simulink library "vmc"  (R2021b)
settings: Solver=VariableStepAuto  StartTime=0.0  StopTime=10.0  RelTol=1e-3
undefined symbols (not defined in the file or in its folder): AVMC_ACCDeltaTqIGain4OVRD_X_kph, AVMC_ACCDeltaTqIGain4OVRD_Y_mps2, AVMC_ACCDeltaTqIGain_X_kph, AVMC_ACCDeltaTqIGain_Y_mps2, AVMC_ACCDeltaTqPGain_X_kph, AVMC_ACCDeltaTqPGain_Y_kph, AVMC_ACCLongSteadyCtrl_X_kph, AVMC_ADSPosGFBDeltaTq_X_kph, AVMC_ADSPosGFBDeltaTq_Y_mps2, AVMC_AggressJerkPCT4AT_X_kph, AVMC_AggressJerkPCT_X_kph, AVMC_AggressLimitPCT4AT_X_kph, AVMC_AggressLimitPCT_X_kph, AVMC_CCLongSteadyCtrl_X_kph, AVMC_DISCDeltaTqIGain_X_kph, AVMC_DISCDeltaTqIGain_Y_mps2, AVMC_DISCDeltaTqPGain_X_kph, AVMC_DISCDeltaTqPGain_Y_kph, AVMC_ESCRegenOut_X_kph, AVMC_ESCRegenOut_Y_Deg, AVMC_ESCRegenOutEnSpd_X_Deg, AVMC_ISOAccLimit_X_mps, AVMC_ISODecLimit_X_mps, AVMC_ISOJerk_X_mps, AVMC_LatESCRegenOut_X_kph, AVMC_LatESCRegenOut_Y_Deg, AVMC_LongAccDeadZone_X_kph, AVMC_LongAccFiltTsforP2_X_Gps, AVMC_MCPresBaseTq_X_bar, AVMC_MSALongSteadyCtrl_X_kph, AVMC_MSAPedalOvrd_X_kph, AVMC_MSASpdBand_X_kph, AVMC_MSATqDownEndTq_X_kph, AVMC_MSATqDownTime_X_kph, AVMC_OPDDisSlideRate_X_Deg, AVMC_OVRD2ActSR2FCMCMD_X_mps2, AVMC_PedalTqRWhlRatio_X_Nm, AVMC_PedalTqRWhlRatio_Y_gps, AVMC_PedalTqRWhlSlipGain_X_rat, AVMC_PedalTqRWhlSlipGain_Y_kph, AVMC_PedalTqRWhSTRGGain_X_deg, AVMC_PedalTqRWhSTRGGain_Y_kph, AVMC_RDCDetectTime_X_kph, AVMC_RDCDetectTime_Y_pct, AVMC_RDCEnSlideRate_X_Deg, AVMC_RearWhlTqRatio_X_Nm, AVMC_RearWhlTqRatio_Y_gps, AVMC_RearWhlTqSlipGain_X_rat, AVMC_RearWhlTqSlipGain_Y_kph, AVMC_RearWhlTqSTRGGain_X_deg, AVMC_RearWhlTqSTRGGain_Y_kph, AVMC_ReqBrkJoinDecSR_X_mps2, AVMC_SoftJerkPCT_X_kph, AVMC_SoftLimitPCT_X_kph, AVMC_StESCYaw_X_kph, AVMC_StESCYaw_Y_Deg, AVMC_StESCYawCom_X_kph, AVMC_StESCYawCom_Y_Gps, AVMC_TMSpdBaseTq_X_rpm, AVMC_VehHoldDecCtrlTime2_X_kph ... (+411)
libraries: hcu_lib x108, simulink x82, tqr x1, simulink_extras x1
(part 5 of 14)

== system vmc/VMC/VMC/Slide Rate  Calculation ==
  VINP_LFRawWhlSpeed_kph : Inport
  VINP_RFRawWhlSpeed_kph : Inport  Port=2
  VINP_LRRawWhlSpeed_kph : Inport  Port=3
  VINP_RRRawWhlSpeed_kph : Inport  Port=4
  VINP_VehSpeed_kph : Inport  Port=5
  VINP_BrkPedalPos_pct : Inport  Port=6
  VINP_BrkSwSta_flg : Inport  Port=7
  VINP_LongAccel_Gps : Inport  Port=8
  VVMC_LongAcc_Gps : Inport  Port=9
  task_time_s : Inport  Port=10
  VTQD_AfterAvailableTqDemFr_Nm : Inport  Port=11
  VTQD_AfterAvailableTqDemRr_Nm : Inport  Port=12
  VTQD_EquivAccPedalSWSta_flg : Inport  Port=13
  VTQD_GearActualPosn_enum : Inport  Port=14
  VTQD_RegenMode_enum : Inport  Port=15
  VTQD_VehActSpd_kph : Inport  Port=16
  VVMC_EstSlope_Deg : Inport  Port=17
  4Wheel Calculation : Subsystem
  Alternative Wheel Slide Calculation : Subsystem
  Coordination : Subsystem
  Partial Wheel Calculation : Subsystem
  VVMC_RawWhlSpdSlideRate_pct : Outport
  VVMC_LFWhlSpdSlideRate_pct : Outport  Port=2
  VVMC_RFWhlSpdSlideRate_pct : Outport  Port=3
  VVMC_LRWhlSpdSlideRate_pct : Outport  Port=4
  VVMC_RRWhlSpdSlideRate_pct : Outport  Port=5
  VVMC_LF4WhlSpdSlideRate_pct : Outport  Port=6
  VVMC_RF4WhlSpdSlideRate_pct : Outport  Port=7
  VVMC_LR4WhlSpdSlideRate_pct : Outport  Port=8
  VVMC_RR4WhlSpdSlideRate_pct : Outport  Port=9
  VVMC_PredictVehSpd_kph : Outport  Port=10
  VVMC_4WhlSpdSlideRate_pct : Outport  Port=11
  VVMC_ActMaxSlideRate_pct : Outport  Port=12
  VVMC_ActLFSlideRate_pct : Outport  Port=13
  VVMC_ActRFSlideRate_pct : Outport  Port=14
  VVMC_ActLRSlideRate_pct : Outport  Port=15
  VVMC_ActRRSlideRate_pct : Outport  Port=16
  VVMC_AltLWhlSlideRate_pct : Outport  Port=17
  VVMC_AltRWhlSlideRate_pct : Outport  Port=18
  VVMC_AltWhlSlideRate_pct : Outport  Port=19
  wires:
  VINP_BrkSwSta_flg/1 -> [VINP_BrkSwSta_flg]
  VTQD_AfterAvailableTqDemFr_Nm/1 -> [VTQD_AfterAvailableTqDemFr_Nm]
  [VVMC_RF4WhlSpdSlideRate_pct] -> VVMC_RF4WhlSpdSlideRate_pct/1
  [VVMC_ActRRSlideRate_pct] -> VVMC_ActRRSlideRate_pct/1
  VTQD_EquivAccPedalSWSta_flg/1 -> [VTQD_EquivAccPedalSWSta_flg]
  [VVMC_LFWhlSpdSlideRate_pct] -> VVMC_LFWhlSpdSlideRate_pct/1
  VINP_BrkPedalPos_pct/1 -> [VINP_BrkPedalPos_pct]
  [VVMC_RRWhlSpdSlideRate_pct] -> VVMC_RRWhlSpdSlideRate_pct/1
  task_time_s/1 -> [task_time_s]
  VINP_RRRawWhlSpeed_kph/1 -> [VINP_RRRawWhlSpeed_kph]
  [VVMC_ActMaxSlideRate_pct] -> VVMC_ActMaxSlideRate_pct/1
  [VVMC_RFWhlSpdSlideRate_pct] -> VVMC_RFWhlSpdSlideRate_pct/1
  [VVMC_LR4WhlSpdSlideRate_pct] -> VVMC_LR4WhlSpdSlideRate_pct/1
  [VVMC_ActRFSlideRate_pct] -> VVMC_ActRFSlideRate_pct/1
  [VVMC_RR4WhlSpdSlideRate_pct] -> VVMC_RR4WhlSpdSlideRate_pct/1
  VINP_RFRawWhlSpeed_kph/1 -> [VINP_RFRawWhlSpeed_kph]
  VINP_VehSpeed_kph/1 -> [VINP_VehSpeed_kph]
  [VVMC_ActLRSlideRate_pct] -> VVMC_ActLRSlideRate_pct/1
  [VVMC_PredictVehSpd_kph] -> VVMC_PredictVehSpd_kph/1
  VINP_LRRawWhlSpeed_kph/1 -> [VINP_LRRawWhlSpeed_kph]
  [VVMC_LF4WhlSpdSlideRate_pct] -> VVMC_LF4WhlSpdSlideRate_pct/1
  [VVMC_RawWhlSpdSlideRate_pct] -> VVMC_RawWhlSpdSlideRate_pct/1
  VINP_LFRawWhlSpeed_kph/1 -> [VINP_LFRawWhlSpeed_kph]
  [VVMC_LRWhlSpdSlideRate_pct] -> VVMC_LRWhlSpdSlideRate_pct/1
  [VVMC_ActLFSlideRate_pct] -> VVMC_ActLFSlideRate_pct/1
  [VVMC_4WhlSpdSlideRate_pct] -> VVMC_4WhlSpdSlideRate_pct/1
  VVMC_LongAcc_Gps/1 -> [VVMC_LongAcc_Gps]
  VTQD_AfterAvailableTqDemRr_Nm/1 -> [VTQD_AfterAvailableTqDemRr_Nm]
  [VINP_LFRawWhlSpeed_kph] -> Alternative Wheel Slide Calculation/1(VINP_LFRawWhlSpeed_kph)
  [VINP_RFRawWhlSpeed_kph] -> Alternative Wheel Slide Calculation/2(VINP_RFRawWhlSpeed_kph)
  [VINP_LRRawWhlSpeed_kph] -> Alternative Wheel Slide Calculation/3(VINP_LRRawWhlSpeed_kph)
  [VINP_RRRawWhlSpeed_kph] -> Alternative Wheel Slide Calculation/4(VINP_RRRawWhlSpeed_kph)
  Alternative Wheel Slide Calculation/1(VVMC_AltLWhlSlideRate_pct) -> [VVMC_AltLWhlSlideRate_pct]
  Alternative Wheel Slide Calculation/2(VVMC_AltRWhlSlideRate_pct) -> [VVMC_AltRWhlSlideRate_pct]
  Alternative Wheel Slide Calculation/3(VVMC_AltWhlSlideRate_pct) -> [VVMC_AltWhlSlideRate_pct]
  [VVMC_AltLWhlSlideRate_pct] -> VVMC_AltLWhlSlideRate_pct/1
  [VVMC_AltRWhlSlideRate_pct] -> VVMC_AltRWhlSlideRate_pct/1
  [VVMC_AltWhlSlideRate_pct] -> VVMC_AltWhlSlideRate_pct/1
  Partial Wheel Calculation/2(VVMC_LFWhlSpdSlideRate_pct) -> [VVMC_LFWhlSpdSlideRate_pct]
  Partial Wheel Calculation/5(VVMC_RRWhlSpdSlideRate_pct) -> [VVMC_RRWhlSpdSlideRate_pct]
  Partial Wheel Calculation/3(VVMC_RFWhlSpdSlideRate_pct) -> [VVMC_RFWhlSpdSlideRate_pct]
  Partial Wheel Calculation/1(VVMC_RawWhlSpdSlideRate_pct) -> [VVMC_RawWhlSpdSlideRate_pct]
  [VINP_RFRawWhlSpeed_kph] -> Partial Wheel Calculation/2(VINP_RFRawWhlSpeed_kph)
  [VINP_LRRawWhlSpeed_kph] -> Partial Wheel Calculation/3(VINP_LRRawWhlSpeed_kph)
  [VTQD_AfterAvailableTqDemFr_Nm] -> Partial Wheel Calculation/5(VTQD_AfterAvailableTqDemFr_Nm)
  [VINP_LFRawWhlSpeed_kph] -> Partial Wheel Calculation/1(VINP_LFRawWhlSpeed_kph)
  [VINP_RRRawWhlSpeed_kph] -> Partial Wheel Calculation/4(VINP_RRRawWhlSpeed_kph)
  [VTQD_AfterAvailableTqDemRr_Nm] -> Partial Wheel Calculation/6(VTQD_AfterAvailableTqDemRr_Nm)
  Partial Wheel Calculation/4(VVMC_LRWhlSpdSlideRate_pct) -> [VVMC_LRWhlSpdSlideRate_pct]
  4Wheel Calculation/3(VVMC_LR4WhlSpdSlideRate_pct) -> [VVMC_LR4WhlSpdSlideRate_pct]
  [task_time_s] -> 4Wheel Calculation/6(task_time_s)
  4Wheel Calculation/1(VVMC_LF4WhlSpdSlideRate_pct) -> [VVMC_LF4WhlSpdSlideRate_pct]
  4Wheel Calculation/7(VVMC_AllWhlSkid_flg) -> [VVMC_AllWhlSkid_flg]
  [VVMC_LongAcc_Gps] -> 4Wheel Calculation/5(VVMC_LongAcc_Gps)
  4Wheel Calculation/4(VVMC_RR4WhlSpdSlideRate_pct) -> [VVMC_RR4WhlSpdSlideRate_pct]
  [VTQD_AfterAvailableTqDemRr_Nm] -> 4Wheel Calculation/9(VTQD_AfterAvailableTqDemRr_Nm)
  [VTQD_AfterAvailableTqDemFr_Nm] -> 4Wheel Calculation/8(VTQD_AfterAvailableTqDemFr_Nm)
  [VINP_VehSpeed_kph] -> 4Wheel Calculation/7(VINP_VehSpeed_kph)
  4Wheel Calculation/5(VVMC_PredictVehSpd_kph) -> [VVMC_PredictVehSpd_kph]
  [VINP_LRRawWhlSpeed_kph] -> 4Wheel Calculation/3(VINP_LRRawWhlSpeed_kph)
  [VINP_RRRawWhlSpeed_kph] -> 4Wheel Calculation/4(VINP_RRRawWhlSpeed_kph)
  [VINP_LFRawWhlSpeed_kph] -> 4Wheel Calculation/1(VINP_LFRawWhlSpeed_kph)
  [VINP_RFRawWhlSpeed_kph] -> 4Wheel Calculation/2(VINP_RFRawWhlSpeed_kph)
  4Wheel Calculation/2(VVMC_RF4WhlSpdSlideRate_pct) -> [VVMC_RF4WhlSpdSlideRate_pct]
  4Wheel Calculation/6(VVMC_4WhlSpdSlideRate_pct) -> [VVMC_4WhlSpdSlideRate_pct]
  [VVMC_LF4WhlSpdSlideRate_pct] -> Coordination/14(VVMC_LF4WhlSpdSlideRate_pct)
  [VVMC_RR4WhlSpdSlideRate_pct] -> Coordination/17(VVMC_RR4WhlSpdSlideRate_pct)
  [VVMC_LR4WhlSpdSlideRate_pct] -> Coordination/16(VVMC_LR4WhlSpdSlideRate_pct)
  [task_time_s] -> Coordination/6(task_time_s)
  [VVMC_LFWhlSpdSlideRate_pct] -> Coordination/9(VVMC_LFWhlSpdSlideRate_pct)
  [VTQD_AfterAvailableTqDemFr_Nm] -> Coordination/1(VTQD_AfterAvailableTqDemFr_Nm)
  [VVMC_AltWhlSlideRate_pct] -> Coordination/20(VVMC_AltWhlSlideRate_pct)
  [VVMC_RFWhlSpdSlideRate_pct] -> Coordination/10(VVMC_RFWhlSpdSlideRate_pct)
  [VTQD_EquivAccPedalSWSta_flg] -> Coordination/2(VTQD_EquivAccPedalSWSta_flg)
  [VVMC_AllWhlSkid_flg] -> Coordination/18(VVMC_AllWhlSkid_flg)
  [VVMC_4WhlSpdSlideRate_pct] -> Coordination/13(VVMC_4WhlSpdSlideRate_pct)
  [VINP_VehSpeed_kph] -> Coordination/5(VINP_VehSpeed_kph)
  Coordination/3(VVMC_ActRFSlideRate_pct) -> [VVMC_ActRFSlideRate_pct]
  [VVMC_RawWhlSpdSlideRate_pct] -> Coordination/8(VVMC_RawWhlSpdSlideRate_pct)
  [VTQD_AfterAvailableTqDemRr_Nm] -> Coordination/19(VTQD_AfterAvailableTqDemRr_Nm)
  Coordination/4(VVMC_ActLRSlideRate_pct) -> [VVMC_ActLRSlideRate_pct]
  [VVMC_PredictVehSpd_kph] -> Coordination/4(VVMC_PredictVehSpd_kph)
  [VINP_BrkSwSta_flg] -> Coordination/7(VINP_BrkSwSta_flg)
  [VVMC_LRWhlSpdSlideRate_pct] -> Coordination/11(VVMC_LRWhlSpdSlideRate_pct)
  [VVMC_RRWhlSpdSlideRate_pct] -> Coordination/12(VVMC_RRWhlSpdSlideRate_pct)
  [VINP_BrkPedalPos_pct] -> Coordination/3(VINP_BrkPedalPos_pct)
  Coordination/1(VVMC_ActMaxSlideRate_pct) -> [VVMC_ActMaxSlideRate_pct]
  Coordination/5(VVMC_ActRRSlideRate_pct) -> [VVMC_ActRRSlideRate_pct]
  Coordination/2(VVMC_ActLFSlideRate_pct) -> [VVMC_ActLFSlideRate_pct]
  [VVMC_RF4WhlSpdSlideRate_pct] -> Coordination/15(VVMC_RF4WhlSpdSlideRate_pct)
  [VTQD_GearActualPosn_enum] -> 4Wheel Calculation/10(VTQD_GearActualPosn_enum)
  VTQD_GearActualPosn_enum/1 -> [VTQD_GearActualPosn_enum]
  VINP_LongAccel_Gps/1 -> [VINP_LongAccel_Gps]
  [VINP_LongAccel_Gps] -> 4Wheel Calculation/11(VINP_LongAccel_Gps)
  VVMC_EstSlope_Deg/1 -> [VVMC_EstSlope_Deg]
  VTQD_RegenMode_enum/1 -> [VTQD_RegenMode_enum]
  VTQD_VehActSpd_kph/1 -> [VTQD_VehActSpd_kph]
  [VTQD_RegenMode_enum] -> Coordination/22(VTQD_RegenMode_enum)
  [VTQD_VehActSpd_kph] -> Coordination/21(VTQD_VehActSpd_kph)
  [VVMC_EstSlope_Deg] -> Coordination/23(VVMC_EstSlope_Deg)

== system vmc/VMC/VMC/SpeedArbitration ==
  VVMC_VMCCCCtrlAvail_flg : Inport
  VVMC_VMCMSACtrlAvail_flg : Inport  Port=2
  VVMC_VMCACCCtrlAvail_flg : Inport  Port=3
  VVMC_VMCAEBCtrlAvail_flg : Inport  Port=4
  VINP_ADASAEBReq_enum : Inport  Port=5
  VINP_ADASAEBSta_enum : Inport  Port=6
  VDSC_DISCSta_enum : Inport  Port=7
  VINP_ADASACCSta_enum : Inport  Port=8
  VVMC_CCCtrlSta_enum : Inport  Port=9
  VVMC_MSACtrlSta_enum : Inport  Port=10
  VDSC_DISCTargetSpd_kph : Inport  Port=11
  VVMC_FeatSetSpdForCalcu_kph : Inport  Port=12
  VDSC_DISCTurn_flg : Inport  Port=13
  VVMC_MeterIndSpeedForCalcu_kph : Inport  Port=14
  VINP_VehSpeed_kph : Inport  Port=15
  VDSC_AccDecResp_flg : Inport  Port=16
  VDSC_AutoTurnMode_flg : Inport  Port=17
  VVMC_AntiSpdLimSpdEn_flg : Inport  Port=18
  VVMC_AntiLimitSpd_kph : Inport  Port=19
  VDSC_PreACC_flg : Inport  Port=20
  AND : Logic  AllPortsSameDT=off  OutDataTypeStr=boolean
  AND1 : Logic  AllPortsSameDT=off  OutDataTypeStr=boolean
  Cast To Single : DataTypeConversion  OutDataTypeStr=uint8
  Cast To Single1 : DataTypeConversion  OutDataTypeStr=uint8
  Cast To Single2 : DataTypeConversion  OutDataTypeStr=single
  Cast To Single3 : DataTypeConversion  OutDataTypeStr=single
  Cast To Single4 : DataTypeConversion  OutDataTypeStr=single
  Constant : Constant  Value=KVMC_ExternalCtrlSW_flg
  Constant1 : Constant  Value=KVMC_ExternalCtrlSW_flg
  Constant11 : Constant  Value=KVMC_DISCDecCtrlTest_flg
  Constant12 : Constant  Value=ENUM_DISCSTA_ACTIVE
  Constant13 : Constant  Value=HUNDRED
  Constant14 : Constant  Value=KVMC_DISCDecCtrlTest_flg
  Constant15 : Constant  Value=ENUM_DISCSTA_ACTIVE
  Constant16 : Constant  Value=HUNDRED
  Constant2 : Constant  Value=KVMC_ExternalCtrlSW_flg
  Constant3 : Constant  Value=KVMC_ExternalCtrlSta_enum
  Constant4 : Constant  Value=KVMC_ExternalSpeedTarget_kph
  Constant5 : Constant  Value=KVMC_ExternalCtrlAGSV_flg
  Constant6 : Constant  Value=KVMC_AutoTurnJerkHiGain_pct
  Constant7 : Constant  Value=KVMC_AutoTurnLimitHiGain_pct
  Constant8 : Constant  Value=ENUM_FEATSTACFM_MSA
  Constant9 : Constant  Value=ENUM_FEATSTACFM_MSA
  Divide : Product  Inputs=**
  Divide1 : Product  Inputs=**
  Feature Arbitration : Subsystem
  Feature Status Confirm : Subsystem
  OR : Logic  Operator=OR  Inputs=3  AllPortsSameDT=off  OutDataTypeStr=boolean
  OR1 : Logic  Operator=OR  Inputs=3  AllPortsSameDT=off  OutDataTypeStr=boolean
  Relational Operator : RelationalOperator  Operator===  OutDataTypeStr=boolean  RndMeth=Simplest
  Relational Operator1 : RelationalOperator  Operator===  OutDataTypeStr=boolean  RndMeth=Simplest
  Response Gain : Subsystem
  Round : Rounding  Operator=round
  Switch{,1..9} (10 alike) : Switch  Criteria=u2 > Threshold
  VVMC_FeatArbitrSta_enum : Outport
  VVMC_FeatReqSpd_kph : Outport  Port=2
  VVMC_JerkPCT_pct : Outport  Port=3
  VVMC_LimitPCT_pct : Outport  Port=4
  wires:
  [VINP_VehSpeed_kph] -> Response Gain/5(VINP_VehSpeed_kph)
  VINP_VehSpeed_kph/1 -> [VINP_VehSpeed_kph]
  [VVMC_FeatReqSpd_kph] -> Response Gain/3(VVMC_FeatReqSpd_kph)
  [VVMC_MeterIndSpeedForCalcu_kph] -> Response Gain/4(VVMC_MeterIndSpeedForCalcu_kph)
  VVMC_MeterIndSpeedForCalcu_kph/1 -> [VVMC_MeterIndSpeedForCalcu_kph]
  Round/1 -> Cast To Single2/1
  [VINP_ADASAEBReq_enum] -> Feature Status Confirm/10(VINP_ADASAEBReq_enum)
  VINP_ADASAEBReq_enum/1 -> [VINP_ADASAEBReq_enum]
  [VVMC_VMCCCCtrlAvail_flg] -> Feature Status Confirm/1(VVMC_VMCCCCtrlAvail_flg)
  [VVMC_VMCMSACtrlAvail_flg] -> Feature Status Confirm/2(VVMC_VMCMSACtrlAvail_flg)
  VVMC_VMCCCCtrlAvail_flg/1 -> [VVMC_VMCCCCtrlAvail_flg]
  VVMC_VMCMSACtrlAvail_flg/1 -> [VVMC_VMCMSACtrlAvail_flg]
  [VVMC_VMCAEBCtrlAvail_flg] -> Feature Status Confirm/3(VVMC_VMCAEBCtrlAvail_flg)
  [VVMC_VMCACCCtrlAvail_flg] -> Feature Status Confirm/4(VVMC_VMCACCCtrlAvail_flg)
  VVMC_VMCAEBCtrlAvail_flg/1 -> [VVMC_VMCAEBCtrlAvail_flg]
  VVMC_VMCACCCtrlAvail_flg/1 -> [VVMC_VMCACCCtrlAvail_flg]
  Switch4/1 -> Switch9/3
  Switch3/1 -> Switch8/3
  Switch7/1 -> [VVMC_FeatReqSpd_kph]  "VVMC_FeatReqSpd_kph"
  Switch6/1 -> [VVMC_FeatArbitrSta_enum]  "VVMC_FeatArbitrSta_enum"
  Switch5/1 -> [VVMC_FeatStaConfirm_enum]  "VVMC_FeatStaConfirm_enum"
  [VVMC_JerkPCT_pct] -> VVMC_JerkPCT_pct/1
  [VVMC_LimitPCT_pct] -> VVMC_LimitPCT_pct/1
  Response Gain/1(VVMC_JerkPCT_pct) -> Cast To Single3/1
  Response Gain/2(VVMC_LimitPCT_pct) -> Cast To Single4/1
  [VVMC_FeatArbitrSta_enum] -> Response Gain/2(VVMC_FeatArbitrSta_enum)
  Switch2/1 -> Response Gain/1(VDSC_DISCTurn_flg)
  [VVMC_FeatReqSpd_kph] -> VVMC_FeatReqSpd_kph/1
  [VVMC_FeatArbitrSta_enum] -> VVMC_FeatArbitrSta_enum/1
  Feature Arbitration/2(VVMC_FeatReqSpd_kph) -> Round/1
  Feature Arbitration/1(VVMC_FeatArbitrSta_enum) -> Cast To Single1/1
  [VVMC_FeatSetSpdForCalcu_kph] -> Feature Arbitration/3(VVMC_FeatSetSpdForCalcu_kph)
  [VVMC_FeatStaConfirm_enum] -> Feature Arbitration/1(VVMC_FeatStaConfirm_enum)
  Feature Status Confirm/1(VVMC_FeatStaConfirm_enum) -> Cast To Single/1
  [VVMC_MSACtrlSta_enum] -> Feature Status Confirm/9(VVMC_MSACtrlSta_enum)
  [VVMC_CCCtrlSta_enum] -> Feature Status Confirm/8(VVMC_CCCtrlSta_enum)
  [VINP_ADASACCSta_enum] -> Feature Status Confirm/7(VINP_ADASACCSta_enum)
  Switch/1 -> Feature Status Confirm/6(VDSC_DISCSta_enum)
  [VINP_ADASAEBSta_enum] -> Feature Status Confirm/5(VINP_ADASAEBSta_enum)
  VDSC_DISCTurn_flg/1 -> [VDSC_DISCTurn_flg]
  VVMC_FeatSetSpdForCalcu_kph/1 -> [VVMC_FeatSetSpdForCalcu_kph]
  VDSC_DISCTargetSpd_kph/1 -> [VDSC_DISCTargetSpd_kph]
  VVMC_MSACtrlSta_enum/1 -> [VVMC_MSACtrlSta_enum]
  VVMC_CCCtrlSta_enum/1 -> [VVMC_CCCtrlSta_enum]
  VINP_ADASACCSta_enum/1 -> [VINP_ADASACCSta_enum]
  VDSC_DISCSta_enum/1 -> [VDSC_DISCSta_enum]
  VINP_ADASAEBSta_enum/1 -> [VINP_ADASAEBSta_enum]
  Switch1/1 -> Feature Arbitration/2(VDSC_DISCTargetSpd_kph)
  [VDSC_DISCSta_enum] -> Switch/3
  Constant1/1 -> Switch1/2
  Constant5/1 -> Switch2/1
  [VDSC_DISCTargetSpd_kph] -> Switch1/3
  Constant3/1 -> Switch/1
  Constant2/1 -> Switch2/2
  Constant4/1 -> Switch1/1
  Constant/1 -> Switch/2
  [VDSC_DISCTurn_flg] -> Switch2/3
  VDSC_AccDecResp_flg/1 -> [VDSC_AccDecResp_flg]
  [VDSC_AccDecResp_flg] -> Switch3/2
  Cast To Single3/1 -> Switch3/3, Divide/2
  Constant6/1 -> Divide/1
  Divide/1 -> Switch3/1
  Divide1/1 -> Switch4/1
  Constant7/1 -> Divide1/1
  Cast To Single4/1 -> Divide1/2, Switch4/3
  [VDSC_AccDecResp_flg] -> Switch4/2
  VDSC_AutoTurnMode_flg/1 -> [VDSC_AutoTurnMode_flg]
  [VDSC_AutoTurnMode_flg] -> Response Gain/6(VDSC_AutoTurnMode_flg)
  VVMC_AntiSpdLimSpdEn_flg/1 -> [VVMC_AntiSpdLimSpdEn_flg]
  [VVMC_AntiSpdLimSpdEn_flg] -> Switch5/2
  Cast To Single/1 -> Switch5/3
  Constant8/1 -> Switch5/1
  Constant9/1 -> Switch6/1
  [VVMC_AntiSpdLimSpdEn_flg] -> Switch6/2
  Cast To Single1/1 -> Switch6/3
  [VVMC_AntiSpdLimSpdEn_flg] -> Switch7/2
  Cast To Single2/1 -> Switch7/3
  [VVMC_AntiLimitSpd_kph] -> Switch7/1
  [VDSC_DISCTargetSpd_kph] -> Response Gain/7(VDSC_DISCTargetSpd_kph)
  VVMC_AntiLimitSpd_kph/1 -> [VVMC_AntiLimitSpd_kph]
  VDSC_PreACC_flg/1 -> [VDSC_PreACC_flg]
  AND1/1 -> Switch9/2
  Relational Operator1/1 -> OR1/2
  [VDSC_PreACC_flg] -> OR1/1
  OR1/1 -> AND1/1
  Constant15/1 -> Relational Operator1/2
  [VDSC_DISCSta_enum] -> Relational Operator1/1
  [VDSC_AutoTurnMode_flg] -> OR1/3
  Constant16/1 -> Switch9/1
  Constant14/1 -> AND1/2
  Switch9/1 -> [VVMC_LimitPCT_pct]  "VVMC_LimitPCT_pct"
  [VDSC_DISCSta_enum] -> Relational Operator/1
  Relational Operator/1 -> OR/2
  Constant13/1 -> Switch8/1
  [VDSC_PreACC_flg] -> OR/1
  Constant12/1 -> Relational Operator/2
  Constant11/1 -> AND/2
  [VDSC_AutoTurnMode_flg] -> OR/3
  OR/1 -> AND/1
  AND/1 -> Switch8/2
  Switch8/1 -> [VVMC_JerkPCT_pct]  "VVMC_JerkPCT_pct"
  [VDSC_PreACC_flg] -> Feature Status Confirm/11(VDSC_PreACC_flg)
  [VDSC_PreACC_flg] -> Feature Arbitration/4(VDSC_PreACC_flg)

== system vmc/VMC/VMC/SpeedCalculation ==
  VINP_MeterIndVehSpeed_kph : Inport
  VINP_Distanceunit_flg : Inport  Port=2
  VINP_VehSpeed_kph : Inport  Port=3
  VTQD_VehActSpd_kph : Inport  Port=4
  VDDM_VMCESC1Err_flg : Inport  Port=5
  VDDM_VMCESC5Err_flg : Inport  Port=6
  function : TriggerPort  TriggerType=function-call  VariantControl=(inherit)
  Add4 : Sum
  Add8 : Sum
  Cast To Single1 : DataTypeConversion  OutDataTypeStr=uint8
  Cast To Single{2..3,6..7,10..12} (7 alike) : DataTypeConversion  OutDataTypeStr=single
  Cast To Single13 : DataTypeConversion  OutDataTypeStr=uint8
  Constant1 : Constant  Value=KVMC_MeterSpdRoundSW_flg
  Constant11 : Constant  Value=KPH2MPH
  Constant16 : Constant  Value=KVMC_Veh2MeterSpdFactor_enum
  Constant19 : Constant  Value=KPH2MPH
  Constant2 : Constant  Value=KVMC_MeterSpdRoundSW_flg
  Constant22 : Constant  Value=C_TASK_10MS_S
  Constant23 : Constant  Value=KVMC_MeterSpdBWFilter_raw32
  Constant28 : Constant  Value=KVMC_Veh2MeterSpdLoFactor_enum
  Constant3 : Constant  Value=ONE_INT
  Constant4 : Constant  Value=ONE_INT
  Constant5 : Constant  Value=KVMC_MeterSpdRollAveLevel_enum
  Constant6 : Constant  Value=256
  Constant7 : Constant  Value=ZERO_FLOAT
  Constant8 : Constant  Value=KVMC_Veh2MeterSpdOffset_enum
  Constant9 : Constant  Value=256
  Divide{,2,5,8} (4 alike) : Product  Inputs=**
  FirstOrderFilter6 : hcu_lib/Basic_Blocks/FirstOrderFilter
  Min : MinMax  Function=max  Inputs=2
  OR : Logic  Operator=OR  AllPortsSameDT=off  OutDataTypeStr=boolean
  OR1 : Logic  Operator=OR  AllPortsSameDT=off  OutDataTypeStr=boolean
  Relational Operator : RelationalOperator  Operator=>  OutDataTypeStr=boolean  RndMeth=Simplest
  Relational Operator1 : RelationalOperator  Operator=>  OutDataTypeStr=boolean  RndMeth=Simplest
  RollingAverage : Stateflow chart  TreatAsAtomicUnit=on
  Round : Rounding
  Round1 : Rounding  Operator=round
  Round2 : Rounding
  Round3 : Rounding  Operator=round
  Switch : Switch  Criteria=u2 > Threshold
  Switch1 : Switch  Criteria=u2 > Threshold  Threshold=KVMC_Veh2MeterSpdLoBdy_kph
  Switch2 : Switch  Criteria=u2 > Threshold
  u2 > 0 (1) : Switch  Criteria=u2 > Threshold
  u2 > 0 (1)1 : Switch  Criteria=u2 > Threshold
  u2 > 0 (1)2 : Switch  Criteria=u2 > Threshold
  VVMC_MeterIndSpeed_raw32 : Outport
  VVMC_VehicleSpeed_mph : Outport  Port=2
  VVMC_VehicleSpeed_kph : Outport  Port=3
  VVMC_MeterIndSpeedForCalcu_kph : Outport  Port=4
  wires:
  u2 > 0 (1)/1 -> Cast To Single6/1
  VINP_Distanceunit_flg/1 -> [VINP_Distanceunit_flg]
  [VINP_Distanceunit_flg] -> u2 > 0 (1)/2
  FirstOrderFilter6/1 -> [VVMC_MeterSpdRollAve_kph]  "VVMC_MeterSpdRollAve_kph"
  [VVMC_MeterIndSpeed_raw32] -> VVMC_MeterIndSpeed_raw32/1
  Constant19/1 -> Divide/2
  u2 > 0 (1)2/1 -> [VVMC_MeterIndSpeedForCalcu_kph]  "VVMC_MeterIndSpeedForCalcu_kph"
  [VVMC_VehicleSpeed_kph] -> VVMC_VehicleSpeed_kph/1
  Cast To Single6/1 -> Round1/1, Round/1
  Constant11/1 -> Divide2/2
  Cast To Single2/1 -> Divide2/1
  [VVMC_MeterIndSpeedForCalcu_kph] -> VVMC_MeterIndSpeedForCalcu_kph/1
  u2 > 0 (1)1/1 -> [VVMC_MeterIndSpeed_raw32]  "VVMC_MeterIndSpeed_raw32"
  VINP_VehSpeed_kph/1 -> [VINP_VehSpeed_kph]
  Divide/1 -> u2 > 0 (1)/1
  [VVMC_MeterSpdRollAve_kph] -> Cast To Single7/1, u2 > 0 (1)/3, Round2/1, Round3/1  "VVMC_MeterSpdRollAve_kph"
  Switch2/1 -> Cast To Single10/1, Cast To Single2/1
  Cast To Single7/1 -> Divide/1
  VINP_MeterIndVehSpeed_kph/1 -> [VINP_MeterIndVehSpeed_kph]
  Divide2/1 -> [VVMC_VehicleSpeed_mph]  "VVMC_VehicleSpeed_mph"
  Cast To Single10/1 -> [VVMC_VehicleSpeed_kph]  "VVMC_VehicleSpeed_kph"
  [VVMC_VehicleSpeed_mph] -> VVMC_VehicleSpeed_mph/1
  Constant22/1 -> Add8/1, FirstOrderFilter6/2
  Add8/1 -> FirstOrderFilter6/3
  Constant23/1 -> Add8/2
  Cast To Single3/1 -> FirstOrderFilter6/1
  Constant1/1 -> u2 > 0 (1)1/2
  Round/1 -> u2 > 0 (1)1/3
  Round1/1 -> u2 > 0 (1)1/1
  Round2/1 -> u2 > 0 (1)2/3
  Constant2/1 -> u2 > 0 (1)2/2
  Round3/1 -> u2 > 0 (1)2/1
  RollingAverage/1(VVMC_RollAve_kph) -> Cast To Single3/1
  Constant5/1 -> Cast To Single1/1
  Switch/1 -> Cast To Single12/1
  Constant4/1 -> Cast To Single13/1
  Constant7/1 -> Cast To Single11/1
  Cast To Single12/1 -> RollingAverage/4(VINP_RawData_kph)
  Cast To Single13/1 -> RollingAverage/3(ONE_INT)
  Cast To Single11/1 -> RollingAverage/2(ZERO_FLOAT)
  Cast To Single1/1 -> Min/1
  Min/1 -> RollingAverage/1(KVMC_RollAveLevel_enum)
  Constant3/1 -> Min/2
  VTQD_VehActSpd_kph/1 -> [VTQD_VehActSpd_kph]
  VDDM_VMCESC1Err_flg/1 -> [VDDM_VMCESC1Err_flg]
  VDDM_VMCESC5Err_flg/1 -> [VDDM_VMCESC5Err_flg]
  [VINP_MeterIndVehSpeed_kph] -> Relational Operator/1
  Constant6/1 -> Relational Operator/2
  Relational Operator/1 -> OR/1
  [VDDM_VMCESC5Err_flg] -> OR/2
  Constant28/1 -> Divide8/2
  Switch1/1 -> Switch/1
  Constant8/1 -> Add4/1
  Add4/1 -> Switch1/1
  Divide8/1 -> Switch1/3
  Constant16/1 -> Divide5/1
  Divide5/1 -> Add4/2
  [VTQD_VehActSpd_kph] -> Switch1/2, Divide8/1, Divide5/2
  OR/1 -> Switch/2
  [VINP_MeterIndVehSpeed_kph] -> Switch/3
  OR1/1 -> Switch2/2
  [VDDM_VMCESC1Err_flg] -> OR1/2
  Constant9/1 -> Relational Operator1/2
  Relational Operator1/1 -> OR1/1
  [VINP_VehSpeed_kph] -> Relational Operator1/1
  [VINP_VehSpeed_kph] -> Switch2/3
  [VTQD_VehActSpd_kph] -> Switch2/1

== system vmc/VMC/VMC/Subsystem ==
  VINP_FoxPiCtrlEnSw_flg : Inport
  VINP_FoxPiDIDReseted_flg : Inport  Port=2
  VTQD_GearActualPosn_enum : Inport  Port=3
  VPMM_SysPowerMode_enum : Inport  Port=4
  AND : Logic  Inputs=4  AllPortsSameDT=off  OutDataTypeStr=boolean
  AND1 : Logic  Operator=OR  Inputs=3  AllPortsSameDT=off  OutDataTypeStr=boolean
  AND2 : Logic  Operator=OR  AllPortsSameDT=off  OutDataTypeStr=boolean
  AND3 : Logic  Operator=OR  AllPortsSameDT=off  OutDataTypeStr=boolean
  Constant : Constant  Value=ENUM_GEARACTUALPOSN_P
  Constant1 : Constant  Value=ENUM_PWRSTASW_OFF
  Detect Decrease : simulink/Logic and Bit Operations/Detect Decrease  vinit=0.0  OutDataTypeStr=boolean
  Detect Decrease1 : simulink/Logic and Bit Operations/Detect Decrease  vinit=0.0  OutDataTypeStr=boolean
  Detect Increase{,1..4} (5 alike) : simulink/Logic and Bit Operations/Detect Increase  vinit=0.0  OutDataTypeStr=boolean
  Equal : RelationalOperator  Operator===  OutDataTypeStr=boolean  RndMeth=Simplest
  Equal1 : RelationalOperator  Operator=~=  OutDataTypeStr=boolean  RndMeth=Simplest
  NOT : Logic  Operator=NOT  AllPortsSameDT=off  OutDataTypeStr=boolean
  SR_Latch : hcu_lib/Basic_Blocks/SR_Latch
  SR_Latch1 : hcu_lib/Basic_Blocks/SR_Latch
  SR_Latch2 : hcu_lib/Basic_Blocks/SR_Latch
  VVMC_FoxPiCtrlEnSw_flg : Outport
  wires:
  VINP_FoxPiCtrlEnSw_flg/1 -> [VINP_FoxPiCtrlEnSw_flg]
  [VINP_FoxPiCtrlEnSw_flg] -> Detect Decrease1/1, Detect Increase/1
  [VTQD_GearActualPosn_enum] -> Equal/1
  AND/1 -> SR_Latch/1
  Constant/1 -> Equal/2
  VTQD_GearActualPosn_enum/1 -> [VTQD_GearActualPosn_enum]
  SR_Latch/1 -> VVMC_FoxPiCtrlEnSw_flg/1
  AND1/1 -> SR_Latch/2
  Detect Increase1/1 -> AND1/1
  NOT/1 -> AND1/2
  [VINP_FoxPiCtrlEnSw_flg] -> NOT/1
  VPMM_SysPowerMode_enum/1 -> [VPMM_SysPowerMode_enum]
  [VPMM_SysPowerMode_enum] -> Equal1/1
  Constant1/1 -> Equal1/2
  VINP_FoxPiDIDReseted_flg/1 -> [VINP_FoxPiDIDReseted_flg]
  [VINP_FoxPiDIDReseted_flg] -> AND1/3
  [VINP_FoxPiDIDReseted_flg] -> Detect Decrease/1, Detect Increase3/1
  SR_Latch1/1 -> AND/1
  Detect Decrease/1 -> SR_Latch1/1
  Equal1/1 -> AND/3
  Equal/1 -> [VVMC_GearPosInP_flg]
  [VVMC_GearPosInP_flg] -> Detect Increase1/1
  [VVMC_GearPosInP_flg] -> AND/4
  AND2/1 -> SR_Latch1/2
  [VVMC_GearPosInP_flg] -> Detect Increase2/1
  Detect Increase2/1 -> AND2/2
  Detect Increase3/1 -> AND2/1
  SR_Latch2/1 -> AND/2
  Detect Increase/1 -> SR_Latch2/1
  AND3/1 -> SR_Latch2/2
  Detect Decrease1/1 -> AND3/1
  [VVMC_GearPosInP_flg] -> Detect Increase4/1
  Detect Increase4/1 -> AND3/2

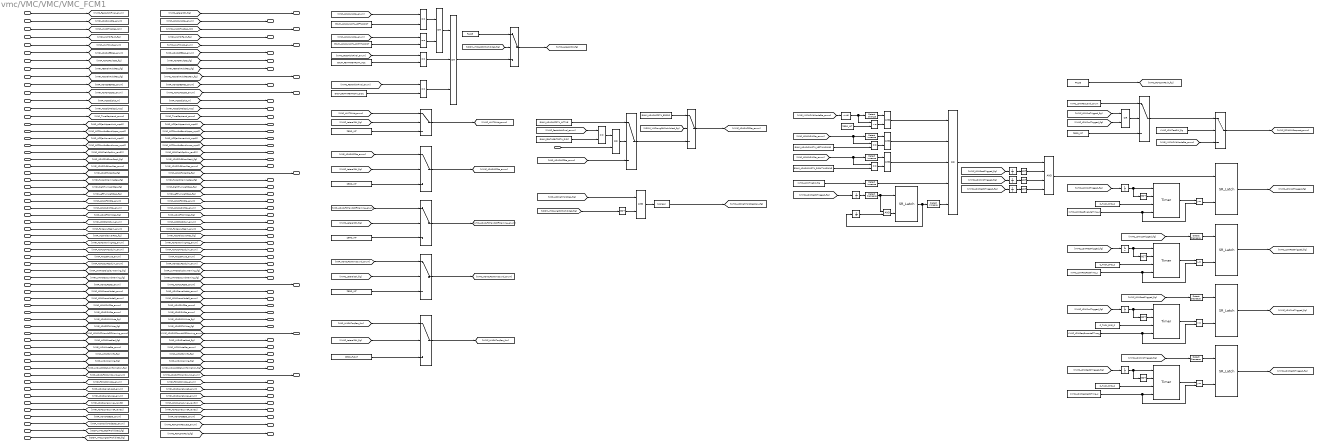
== system vmc/VMC/VMC/VMC_FCM1 ==
  VVMC_FeatArbitrFinal_enum : Inport
  VINP_ADASLKASta_enum : Inport  Port=2
  VINP_LKAStrToqReq_Nm : Inport  Port=3
  VINP_LKATOIFault_flg : Inport  Port=4
  VINP_LKATOIAct_enum : Inport  Port=5
  VINP_ADASAEBReq_enum : Inport  Port=6
  VINP_ADASFaultSta_flg : Inport  Port=7
  VINP_AEBVehHoldReq_flg : Inport  Port=8
  VINP_ACCVehHoldReq_flg : Inport  Port=9
  VINP_ADASDBSReq_enum : Inport  Port=10
  VINP_ADASACCSta_enum : Inport  Port=11
  VINP_ACCObjDist_m : Inport  Port=12
  VINP_ACCObjRelSpd_mps : Inport  Port=13
  VINP_TimeGapLevel_enum : Inport  Port=14
  VINP_ACCJerkUpperLimit_mps3 : Inport  Port=15
  VINP_ACCComfortBandUpper_mps2 : Inport  Port=16
  VINP_ACCJerkLowerLimit_mps3 : Inport  Port=17
  VINP_ACCComfortBandLower_mps2 : Inport  Port=18
  VINP_ADASVehSpdLim_raw32 : Inport  Port=19
  VINP_ADASShftPosnReqA_flg : Inport  Port=20
  VINP_ADASShftPosnReq_enum : Inport  Port=21
  VINP_ADASForceIdle_flg : Inport  Port=22
  VINP_HazardWarningReq_flg : Inport  Port=23
  VINP_RightTurnLightReq_flg : Inport  Port=24
  VINP_LeftTurnLightReq_flg : Inport  Port=25
  VINP_ADASFCWSta_enum : Inport  Port=26
  VINP_ADASLDWSta_enum : Inport  Port=27
  VINP_ADASFltWrnReq_flg : Inport  Port=28
  VINP_ACCObjDstLvl_enum : Inport  Port=29
  VINP_ForceLowBeam_enum : Inport  Port=30
  VINP_ACCTakeoverReq_flg : Inport  Port=31
  VINP_ADASWarningMsg_enum : Inport  Port=32
  VINP_ADASCAMSpdLim_enum : Inport  Port=33
  VINP_TargetType_enum : Inport  Port=34
  VINP_ADASSLIFSpdLim_enum : Inport  Port=35
  VINP_LKAHODDisplayWarning_flg : Inport  Port=36
  VINP_LKAHODSoundWarning_flg : Inport  Port=37
  VINP_ADASLFCSta_enum : Inport  Port=38
  VINP_ADASLaneModeL_enum : Inport  Port=39
  VINP_ADASLaneModeR_enum : Inport  Port=40
  VINP_ADASSLIFSta_enum : Inport  Port=41
  VINP_ADASISASta_enum : Inport  Port=42
  VINP_ADASLDWMute_flg : Inport  Port=43
  VINP_ADASFCWMute_flg : Inport  Port=44
  VINP_ADASLFCHandsOffWarning_enum : Inport  Port=45
  VINP_LVDADisabled_flg : Inport  Port=46
  VINP_LVDAMuteSta_enum : Inport  Port=47
  VINP_LVDAFailinfo_flg : Inport  Port=48
  VINP_LVDAWarning_flg : Inport  Port=49
  VINP_LVDAACCStatusInformation_flg : Inport  Port=50
  VINP_ADASLFCWarnSound_enum : Inport  Port=51
  VINP_FCMACCmode_enum : Inport  Port=52
  VINP_ADASLanetypeR_enum : Inport  Port=53
  VINP_ADASLanetypeL_enum : Inport  Port=54
  VINP_ADASLanecurveL_raw32 : Inport  Port=55
  VINP_ADASLanecurveR_raw32 : Inport  Port=56
  VINP_ADASAEBSta_enum : Inport  Port=57
  VVMC_ACCShutOffHold_flg : Inport  Port=58
  VINP_IVISWCVibModeSta_enum : Inport  Port=59
  VDDM_VMCLatCtrlProhibited_flg : Inport  Port=60
  VDDM_VMCLongCtrlProhibited_flg : Inport  Port=61
  AND1 : Logic  Inputs=4  AllPortsSameDT=off  OutDataTypeStr=boolean
  AND{2..5} (4 alike) : Logic  AllPortsSameDT=off  OutDataTypeStr=boolean
  Cast To Boolean : DataTypeConversion  OutDataTypeStr=boolean
  Cast To Single : DataTypeConversion  OutDataTypeStr=uint8
  Constant : Constant  Value=ZERO_FLOAT
  Constant{1..3,15..16,35} (6 alike) : Constant  Value=ZERO_INT
  Constant10 : Constant  Value=ENUM_FEATARBITRSTA_DISC
  Constant11 : Constant  Value=ENUM_FEATARBITRSTA_DISC
  Constant12 : Constant  Value=FALSE
  Constant13 : Constant  Value=ENUM_ADASACCSTA_ERROR
  Constant25 : Constant  Value=KVMC_LDWReqExecuteTime_s
  Constant26 : Constant  Value=KVMC_LDWReqRestTime_s
  Constant29 : Constant  Value=FALSE
  Constant{30,33..34,36} (4 alike) : Constant  Value=C_TASK_5MS_S
  Constant31 : Constant  Value=KVMC_LDWReqRest2Time_s
  Constant32 : Constant  Value=KVMC_LDWReqExecute2Time_s
  Constant37 : Constant  Value=ENUM_ADASLDWSTA_LEFTWARNING
  Constant38 : Constant  Value=KVMC_LDWTestSW_flg
  Constant39 : Constant  Value=KVMC_LDWReqLevel_enum
  Constant4 : Constant  Value=ENUM_FEATARBITRSTA_ACC
  Constant5 : Constant  Value=ENUM_ADASLDWSTA_RIGHTWARNING
  Constant6 : Constant  Value=ENUM_ADASLKASTA_LEFTASSIST
  Constant7 : Constant  Value=ENUM_ADASLKASTA_RIGHTASSIST
  Constant8 : Constant  Value=KVMC_LDWTrigSW_flg
  Constant9 : Constant  Value=ENUM_ADASACCSTA_ACTIVE
  Detect Change : simulink/Logic and Bit Operations/Detect Change  vinit=0  OutDataTypeStr=boolean
  Detect Decrease{2..5} (4 alike) : simulink/Logic and Bit Operations/Detect Decrease  vinit=0.0  OutDataTypeStr=boolean
  Detect Increase{2..5} (4 alike) : simulink/Logic and Bit Operations/Detect Increase  vinit=0.0  OutDataTypeStr=boolean
  Logical Operator : Logic  Operator=OR  AllPortsSameDT=off  OutDataTypeStr=boolean
  Logical Operator1 : Logic  Operator=OR  Inputs=3  AllPortsSameDT=off  OutDataTypeStr=boolean
  Logical Operator3 : Logic  AllPortsSameDT=off  OutDataTypeStr=boolean
  NOT{,5..11} (8 alike) : Logic  Operator=NOT  AllPortsSameDT=off  OutDataTypeStr=boolean
  OR1 : Logic  Operator=OR  AllPortsSameDT=off  OutDataTypeStr=boolean
  OR3 : Logic  Operator=OR  AllPortsSameDT=off  OutDataTypeStr=boolean
  OR4 : Logic  Operator=OR  Inputs=5  AllPortsSameDT=off  OutDataTypeStr=boolean
  Relational Operator{,1..4,9..10} (7 alike) : RelationalOperator  Operator===  OutDataTypeStr=boolean  RndMeth=Simplest
  Relational Operator{7..8,11..12} (4 alike) : RelationalOperator  OutDataTypeStr=boolean  RndMeth=Simplest
  Relational Operator5 : RelationalOperator  Operator=~=  OutDataTypeStr=boolean  RndMeth=Simplest
  SR_Latch{3..7} (5 alike) : hcu_lib/Basic_Blocks/SR_Latch
  Switch{1..3,10} (4 alike) : Switch  Criteria=u2 > Threshold
  Timer{3..6} (4 alike) : hcu_lib/Basic_Blocks/Timer
  Unit Delay{5..13} (9 alike) : UnitDelay  SampleTime=-1  HasFrameUpgradeWarning=on
  u2 > 0 : Switch  Criteria=u2 > Threshold
  u2 > 0 (1) : Switch  Criteria=u2 > Threshold
  u2 > 0 (2){,2..4} (4 alike) : Switch  Criteria=u2 > Threshold
  VVMC_LateralCtrl_flg : Outport
  VVMC_ADASLKASta_enum : Outport  Port=2
  VVMC_LKAStrToqReq_Nm : Outport  Port=3
  VVMC_LKATOIFault_flg : Outport  Port=4
  VVMC_LKATOIAct_enum : Outport  Port=5
  VVMC_ADASAEBReq_enum : Outport  Port=6
  VVMC_ADASFaultSta_flg : Outport  Port=7
  VVMC_AEBVehHoldReq_flg : Outport  Port=8
  VVMC_ACCVehHoldReqRaw_flg : Outport  Port=9
  VVMC_ADASDBSReq_enum : Outport  Port=10
  VVMC_ADASACCSta_enum : Outport  Port=11
  VVMC_ACCObjDist_m : Outport  Port=12
  VVMC_ACCObjRelSpd_mps : Outport  Port=13
  VVMC_TimeGapLevel_enum : Outport  Port=14
  VVMC_ACCJerkUpperLimit_mps3 : Outport  Port=15
  VVMC_ACCComfortBandUpper_mps2 : Outport  Port=16
  VVMC_ACCJerkLowerLimit_mps3 : Outport  Port=17
  VVMC_ACCComfortBandLower_mps2 : Outport  Port=18
  VVMC_ADASVehSpdLim_raw32 : Outport  Port=19
  VVMC_ADASShftPosnReqA_flg : Outport  Port=20
  VVMC_ADASShftPosnReq_enum : Outport  Port=21
  VVMC_ADASForceIdle_flg : Outport  Port=22
  VVMC_HazardWarningReq_flg : Outport  Port=23
  VVMC_RightTurnLightReq_flg : Outport  Port=24
  VVMC_LeftTurnLightReq_flg : Outport  Port=25
  VVMC_ADASFCWSta_enum : Outport  Port=26
  VVMC_ADASLDWSta_enum : Outport  Port=27
  VVMC_ADASFltWrnReq_flg : Outport  Port=28
  VVMC_ACCObjDstLvl_enum : Outport  Port=29
  VVMC_ForceLowBeam_enum : Outport  Port=30
  VVMC_ACCTakeoverReq_flg : Outport  Port=31
  VVMC_ADASWarningMsg_enum : Outport  Port=32
  VVMC_ADASCAMSpdLim_enum : Outport  Port=33
  VVMC_TargetType_enum : Outport  Port=34
  VVMC_ADASSLIFSpdLim_enum : Outport  Port=35
  VVMC_LKAHODDisplayWarning_flg : Outport  Port=36
  VVMC_LKAHODSoundWarning_flg : Outport  Port=37
  VVMC_ADASLFCSta_enum : Outport  Port=38
  VVMC_ADASLaneModeL_enum : Outport  Port=39
  VVMC_ADASLaneModeR_enum : Outport  Port=40
  VVMC_ADASSLIFSta_enum : Outport  Port=41
  VVMC_ADASISASta_enum : Outport  Port=42
  VVMC_ADASLDWMute_flg : Outport  Port=43
  VVMC_ADASFCWMute_flg : Outport  Port=44
  VVMC_ADASLFCHandsOffWarning_enum : Outport  Port=45
  VVMC_LVDADisabled_flg : Outport  Port=46
  VVMC_LVDAMuteSta_enum : Outport  Port=47
  VVMC_LVDAFailinfo_flg : Outport  Port=48
  VVMC_LVDAWarning_flg : Outport  Port=49
  VVMC_LVDAACCStatusInformation_flg : Outport  Port=50
  VVMC_ADASLFCWarnSound_enum : Outport  Port=51
  VVMC_FCMACCmode_enum : Outport  Port=52
  VVMC_ADASLanetypeR_enum : Outport  Port=53
  VVMC_ADASLanetypeL_enum : Outport  Port=54
  VVMC_ADASLanecurveL_raw32 : Outport  Port=55
  VVMC_ADASLanecurveR_raw32 : Outport  Port=56
  VVMC_ADASAEBSta_enum : Outport  Port=57
  VVMC_FCMLDWRequest_enum : Outport  Port=58
  VVMC_FCMLDWFault_flg : Outport  Port=59
  wires:
  [VVMC_LateralCtrl_flg] -> VVMC_LateralCtrl_flg/1
  u2 > 0 (1)/1 -> [VVMC_LKATOIAct_enum]  "VVMC_LKATOIAct_enum"
  Constant1/1 -> u2 > 0 (1)/3
  [VVMC_LateralCtrl_flg] -> u2 > 0 (1)/2
  u2 > 0/1 -> [VVMC_LKAStrToqReq_Nm]  "VVMC_LKAStrToqReq_Nm"
  Constant/1 -> u2 > 0/3
  [VVMC_LateralCtrl_flg] -> u2 > 0/2
  Switch10/1 -> [VVMC_LateralCtrl_flg]  "VVMC_LateralCtrl_flg"
  Relational Operator3/1 -> Logical Operator1/2
  Logical Operator/1 -> Logical Operator1/1
  Relational Operator2/1 -> Logical Operator/2
  Relational Operator1/1 -> Logical Operator/1
  [VINP_ADASLKASta_enum] -> Relational Operator2/1  "VINP_ADASLKASta_enum"
  [VINP_ADASLKASta_enum] -> Relational Operator1/1  "VINP_ADASLKASta_enum"
  [VVMC_FeatArbitrFinal_enum] -> Relational Operator3/1
  Constant4/1 -> Relational Operator3/2
  Constant6/1 -> Relational Operator1/2
  Constant7/1 -> Relational Operator2/2
  [VINP_LKATOIAct_enum] -> u2 > 0 (1)/1  "VINP_LKATOIAct_enum"
  VINP_LKATOIAct_enum/1 -> [VINP_LKATOIAct_enum]
  VINP_LKATOIFault_flg/1 -> [VINP_LKATOIFault_flg]
  VINP_LKAStrToqReq_Nm/1 -> [VINP_LKAStrToqReq_Nm]
  VINP_ADASLKASta_enum/1 -> [VINP_ADASLKASta_enum]
  VVMC_FeatArbitrFinal_enum/1 -> [VVMC_FeatArbitrFinal_enum]
  VINP_ADASFaultSta_flg/1 -> [VINP_ADASFaultSta_flg]
  VINP_ADASAEBReq_enum/1 -> [VINP_ADASAEBReq_enum]
  VINP_AEBVehHoldReq_flg/1 -> [VINP_AEBVehHoldReq_flg]
  VINP_ADASDBSReq_enum/1 -> [VINP_ADASDBSReq_enum]
  VINP_ACCVehHoldReq_flg/1 -> [VINP_ACCVehHoldReq_flg]
  [VINP_ADASACCSta_enum] -> u2 > 0 (2)/3
  Switch1/1 -> [VVMC_ADASACCSta_enum]  "VVMC_ADASACCSta_enum"
  [VVMC_FeatArbitrFinal_enum] -> Relational Operator/1
  VINP_ADASACCSta_enum/1 -> [VINP_ADASACCSta_enum]
  Constant9/1 -> u2 > 0 (2)/1
  Constant10/1 -> Relational Operator/2
  Relational Operator/1 -> OR1/1
  VINP_ACCJerkUpperLimit_mps3/1 -> [VINP_ACCJerkUpperLimit_mps3]
  VINP_ForceLowBeam_enum/1 -> [VINP_ForceLowBeam_enum]
  VINP_ADASLFCSta_enum/1 -> [VINP_ADASLFCSta_enum]
  VINP_ADASLanecurveR_raw32/1 -> [VINP_ADASLanecurveR_raw32]
  VINP_ADASLDWSta_enum/1 -> [VINP_ADASLDWSta_enum]
  VINP_ADASLaneModeR_enum/1 -> [VINP_ADASLaneModeR_enum]
  VINP_ACCComfortBandLower_mps2/1 -> [VINP_ACCComfortBandLower_mps2]
  VINP_ADASLanecurveL_raw32/1 -> [VINP_ADASLanecurveL_raw32]
  VINP_TargetType_enum/1 -> [VINP_TargetType_enum]
  VINP_ACCJerkLowerLimit_mps3/1 -> [VINP_ACCJerkLowerLimit_mps3]
  VINP_ADASShftPosnReq_enum/1 -> [VINP_ADASShftPosnReq_enum]
  VINP_ADASSLIFSta_enum/1 -> [VINP_ADASSLIFSta_enum]
  VINP_ADASShftPosnReqA_flg/1 -> [VINP_ADASShftPosnReqA_flg]
  VINP_LVDAMuteSta_enum/1 -> [VINP_LVDAMuteSta_enum]
  VINP_ACCComfortBandUpper_mps2/1 -> [VINP_ACCComfortBandUpper_mps2]
  VINP_FCMACCmode_enum/1 -> [VINP_FCMACCmode_enum]
  VINP_ADASCAMSpdLim_enum/1 -> [VINP_ADASCAMSpdLim_enum]
  VINP_LVDADisabled_flg/1 -> [VINP_LVDADisabled_flg]
  VINP_LKAHODDisplayWarning_flg/1 -> [VINP_LKAHODDisplayWarning_flg]
  VINP_ADASLDWMute_flg/1 -> [VINP_ADASLDWMute_flg]
  VINP_ADASFCWSta_enum/1 -> [VINP_ADASFCWSta_enum]
  VINP_LKAHODSoundWarning_flg/1 -> [VINP_LKAHODSoundWarning_flg]
  VINP_LeftTurnLightReq_flg/1 -> [VINP_LeftTurnLightReq_flg]
  VINP_ADASWarningMsg_enum/1 -> [VINP_ADASWarningMsg_enum]
  VINP_ADASFCWMute_flg/1 -> [VINP_ADASFCWMute_flg]
  VINP_ADASLanetypeL_enum/1 -> [VINP_ADASLanetypeL_enum]
  VINP_ADASFltWrnReq_flg/1 -> [VINP_ADASFltWrnReq_flg]
  VINP_RightTurnLightReq_flg/1 -> [VINP_RightTurnLightReq_flg]
  VINP_ACCTakeoverReq_flg/1 -> [VINP_ACCTakeoverReq_flg]
  VINP_ADASLFCWarnSound_enum/1 -> [VINP_ADASLFCWarnSound_enum]
  VINP_ACCObjDstLvl_enum/1 -> [VINP_ACCObjDstLvl_enum]
  VINP_LVDAFailinfo_flg/1 -> [VINP_LVDAFailinfo_flg]
  VINP_HazardWarningReq_flg/1 -> [VINP_HazardWarningReq_flg]
  VINP_ADASSLIFSpdLim_enum/1 -> [VINP_ADASSLIFSpdLim_enum]
  VINP_LVDAWarning_flg/1 -> [VINP_LVDAWarning_flg]
  VINP_ADASLFCHandsOffWarning_enum/1 -> [VINP_ADASLFCHandsOffWarning_enum]
  VINP_ADASLaneModeL_enum/1 -> [VINP_ADASLaneModeL_enum]
  VINP_ADASLanetypeR_enum/1 -> [VINP_ADASLanetypeR_enum]
  VINP_LVDAACCStatusInformation_flg/1 -> [VINP_LVDAACCStatusInformation_flg]
  VINP_ADASVehSpdLim_raw32/1 -> [VINP_ADASVehSpdLim_raw32]
  VINP_ADASForceIdle_flg/1 -> [VINP_ADASForceIdle_flg]
  VINP_ADASISASta_enum/1 -> [VINP_ADASISASta_enum]
  VINP_ACCObjRelSpd_mps/1 -> [VINP_ACCObjRelSpd_mps]
  VINP_ACCObjDist_m/1 -> [VINP_ACCObjDist_m]
  VINP_TimeGapLevel_enum/1 -> [VINP_TimeGapLevel_enum]
  Cast To Boolean/1 -> [VVMC_ACCVehHoldReqRaw_flg]  "VVMC_ACCVehHoldReqRaw_flg"
  Constant15/1 -> u2 > 0 (2)2/3
  u2 > 0 (2)2/1 -> [VVMC_ADASLFCSta_enum]  "VVMC_ADASLFCSta_enum"
  [VINP_ADASLFCSta_enum] -> u2 > 0 (2)2/1
  [VVMC_LateralCtrl_flg] -> u2 > 0 (2)2/2
  [VVMC_LateralCtrl_flg] -> u2 > 0 (2)3/2
  [VINP_ADASLFCHandsOffWarning_enum] -> u2 > 0 (2)3/1
  u2 > 0 (2)3/1 -> [VVMC_ADASLFCHandsOffWarning_enum]  "VVMC_ADASLFCHandsOffWarning_enum"
  Constant16/1 -> u2 > 0 (2)3/3
  Constant3/1 -> u2 > 0 (2)4/3
  u2 > 0 (2)4/1 -> [VVMC_ADASLFCWarnSound_enum]  "VVMC_ADASLFCWarnSound_enum"
  [VINP_ADASLFCWarnSound_enum] -> u2 > 0 (2)4/1
  [VVMC_LateralCtrl_flg] -> u2 > 0 (2)4/2
  [VINP_ADASLKASta_enum] -> VVMC_ADASLKASta_enum/1  "VVMC_ADASLKASta_enum"
  [VVMC_LKAStrToqReq_Nm] -> VVMC_LKAStrToqReq_Nm/1
  [VINP_LKATOIFault_flg] -> VVMC_LKATOIFault_flg/1  "VVMC_LKATOIFault_flg"
  [VVMC_LKATOIAct_enum] -> VVMC_LKATOIAct_enum/1
  [VINP_ADASAEBReq_enum] -> VVMC_ADASAEBReq_enum/1  "VVMC_ADASAEBReq_enum"
  [VINP_ADASFaultSta_flg] -> VVMC_ADASFaultSta_flg/1  "VVMC_ADASFaultSta_flg"
  [VINP_AEBVehHoldReq_flg] -> VVMC_AEBVehHoldReq_flg/1  "VVMC_AEBVehHoldReq_flg"
  [VVMC_ACCVehHoldReqRaw_flg] -> VVMC_ACCVehHoldReqRaw_flg/1
  [VINP_ADASDBSReq_enum] -> VVMC_ADASDBSReq_enum/1  "VVMC_ADASDBSReq_enum"
  [VVMC_ADASACCSta_enum] -> VVMC_ADASACCSta_enum/1
  [VINP_ACCObjDist_m] -> VVMC_ACCObjDist_m/1  "VVMC_ACCObjDist_m"
  [VINP_ACCObjRelSpd_mps] -> VVMC_ACCObjRelSpd_mps/1  "VVMC_ACCObjRelSpd_mps"
  [VINP_TimeGapLevel_enum] -> VVMC_TimeGapLevel_enum/1  "VVMC_TimeGapLevel_enum"
  [VINP_ACCJerkUpperLimit_mps3] -> VVMC_ACCJerkUpperLimit_mps3/1  "VVMC_ACCJerkUpperLimit_mps3"
  [VINP_ACCComfortBandUpper_mps2] -> VVMC_ACCComfortBandUpper_mps2/1  "VVMC_ACCComfortBandUpper_mps2"
  [VINP_ACCJerkLowerLimit_mps3] -> VVMC_ACCJerkLowerLimit_mps3/1  "VVMC_ACCJerkLowerLimit_mps3"
  [VINP_ACCComfortBandLower_mps2] -> VVMC_ACCComfortBandLower_mps2/1  "VVMC_ACCComfortBandLower_mps2"
  [VINP_ADASVehSpdLim_raw32] -> VVMC_ADASVehSpdLim_raw32/1  "VVMC_ADASVehSpdLim_raw32"
  [VINP_ADASShftPosnReqA_flg] -> VVMC_ADASShftPosnReqA_flg/1  "VVMC_ADASShftPosnReqA_flg"
  [VINP_ADASShftPosnReq_enum] -> VVMC_ADASShftPosnReq_enum/1  "VVMC_ADASShftPosnReq_enum"
  [VINP_ADASForceIdle_flg] -> VVMC_ADASForceIdle_flg/1  "VVMC_ADASForceIdle_flg"
  [VINP_HazardWarningReq_flg] -> VVMC_HazardWarningReq_flg/1  "VVMC_HazardWarningReq_flg"
  [VINP_RightTurnLightReq_flg] -> VVMC_RightTurnLightReq_flg/1  "VVMC_RightTurnLightReq_flg"
  [VINP_LeftTurnLightReq_flg] -> VVMC_LeftTurnLightReq_flg/1  "VVMC_LeftTurnLightReq_flg"
  [VINP_ADASFCWSta_enum] -> VVMC_ADASFCWSta_enum/1  "VVMC_ADASFCWSta_enum"
  [VINP_ADASLDWSta_enum] -> VVMC_ADASLDWSta_enum/1  "VVMC_ADASLDWSta_enum"
  [VINP_ADASFltWrnReq_flg] -> VVMC_ADASFltWrnReq_flg/1  "VVMC_ADASFltWrnReq_flg"
  [VINP_ACCObjDstLvl_enum] -> VVMC_ACCObjDstLvl_enum/1  "VVMC_ACCObjDstLvl_enum"
  [VINP_ForceLowBeam_enum] -> VVMC_ForceLowBeam_enum/1  "VVMC_ForceLowBeam_enum"
  [VINP_ACCTakeoverReq_flg] -> VVMC_ACCTakeoverReq_flg/1  "VVMC_ACCTakeoverReq_flg"
  [VINP_ADASWarningMsg_enum] -> VVMC_ADASWarningMsg_enum/1  "VVMC_ADASWarningMsg_enum"
  [VINP_ADASCAMSpdLim_enum] -> VVMC_ADASCAMSpdLim_enum/1  "VVMC_ADASCAMSpdLim_enum"
  [VINP_TargetType_enum] -> VVMC_TargetType_enum/1  "VVMC_TargetType_enum"
  [VINP_ADASSLIFSpdLim_enum] -> VVMC_ADASSLIFSpdLim_enum/1  "VVMC_ADASSLIFSpdLim_enum"
  [VINP_LKAHODDisplayWarning_flg] -> VVMC_LKAHODDisplayWarning_flg/1  "VVMC_LKAHODDisplayWarning_flg"
  [VINP_LKAHODSoundWarning_flg] -> VVMC_LKAHODSoundWarning_flg/1  "VVMC_LKAHODSoundWarning_flg"
  [VVMC_ADASLFCSta_enum] -> VVMC_ADASLFCSta_enum/1
  [VINP_ADASLaneModeL_enum] -> VVMC_ADASLaneModeL_enum/1  "VVMC_ADASLaneModeL_enum"
  [VINP_ADASLaneModeR_enum] -> VVMC_ADASLaneModeR_enum/1  "VVMC_ADASLaneModeR_enum"
  [VINP_ADASSLIFSta_enum] -> VVMC_ADASSLIFSta_enum/1  "VVMC_ADASSLIFSta_enum"
  [VINP_ADASISASta_enum] -> VVMC_ADASISASta_enum/1  "VVMC_ADASISASta_enum"
  [VINP_ADASLDWMute_flg] -> VVMC_ADASLDWMute_flg/1  "VVMC_ADASLDWMute_flg"
  [VINP_ADASFCWMute_flg] -> VVMC_ADASFCWMute_flg/1  "VVMC_ADASFCWMute_flg"
  [VVMC_ADASLFCHandsOffWarning_enum] -> VVMC_ADASLFCHandsOffWarning_enum/1
  [VINP_LVDADisabled_flg] -> VVMC_LVDADisabled_flg/1  "VVMC_LVDADisabled_flg"
  [VINP_LVDAMuteSta_enum] -> VVMC_LVDAMuteSta_enum/1  "VVMC_LVDAMuteSta_enum"
  [VINP_LVDAFailinfo_flg] -> VVMC_LVDAFailinfo_flg/1  "VVMC_LVDAFailinfo_flg"
  [VINP_LVDAWarning_flg] -> VVMC_LVDAWarning_flg/1  "VVMC_LVDAWarning_flg"
  [VINP_LVDAACCStatusInformation_flg] -> VVMC_LVDAACCStatusInformation_flg/1  "VVMC_LVDAACCStatusInformation_flg"
  [VVMC_ADASLFCWarnSound_enum] -> VVMC_ADASLFCWarnSound_enum/1
  [VINP_FCMACCmode_enum] -> VVMC_FCMACCmode_enum/1  "VVMC_FCMACCmode_enum"
  [VINP_ADASLanetypeR_enum] -> VVMC_ADASLanetypeR_enum/1  "VVMC_ADASLanetypeR_enum"
  [VINP_ADASLanetypeL_enum] -> VVMC_ADASLanetypeL_enum/1  "VVMC_ADASLanetypeL_enum"
  [VINP_ADASLanecurveL_raw32] -> VVMC_ADASLanecurveL_raw32/1  "VVMC_ADASLanecurveL_raw32"
  [VINP_ADASLanecurveR_raw32] -> VVMC_ADASLanecurveR_raw32/1  "VVMC_ADASLanecurveR_raw32"
  VINP_ADASAEBSta_enum/1 -> [VINP_ADASAEBSta_enum]
  [VINP_ADASAEBSta_enum] -> VVMC_ADASAEBSta_enum/1  "VVMC_ADASAEBSta_enum"
  [VVMC_FCMLDWRequest_enum] -> VVMC_FCMLDWRequest_enum/1  "VVMC_FCMLDWRequest_enum"
  [VVMC_FCMLDWFault_flg] -> VVMC_FCMLDWFault_flg/1  "VVMC_FCMLDWFault_flg"
  [VINP_ACCVehHoldReq_flg] -> Logical Operator3/1
  Constant11/1 -> Relational Operator4/2
  [VVMC_FeatArbitrFinal_enum] -> Relational Operator4/1
  Relational Operator4/1 -> Logical Operator1/3
  [VINP_LKAStrToqReq_Nm] -> u2 > 0/1  "VINP_LKAStrToqReq_Nm"
  VVMC_ACCShutOffHold_flg/1 -> OR1/2
  OR1/1 -> u2 > 0 (2)/2
  Timer4/1 -> Relational Operator11/1
  [VINP_ADASLDWSta_enum] -> Relational Operator10/1, Detect Increase5/1  "VVMC_ADASLDWSta_enum"
  Relational Operator10/1 -> AND4/2
  Unit Delay6/1 -> Timer4/1, NOT6/1
  SR_Latch3/1 -> [VVMC_LDW1stTrigged_flg]  "VVMC_LDW1stTrigged_flg"
  [VVMC_LDW1stTrigged_flg] -> Unit Delay5/1
  [VVMC_LDW2ndTrigged_flg] -> Unit Delay7/1
  SR_Latch4/1 -> [VVMC_LDWRestTrigged_flg]  "VVMC_LDWRestTrigged_flg"
  SR_Latch7/1 -> Unit Delay13/1, Detect Increase3/1
  Relational Operator7/1 -> SR_Latch6/2
  Timer6/1 -> Relational Operator7/1
  Constant29/1 -> [VVMC_FCMLDWFault_flg]  "VVMC_FCMLDWFault_flg"
  Timer3/1 -> Relational Operator8/1
  Constant25/1 -> Relational Operator8/2, Timer3/4
  NOT7/1 -> Timer5/2
  Switch2/1 -> [VVMC_FCMLDWRequest_enum]  "VVMC_FCMLDWRequest_enum"
  Constant39/1 -> Switch3/1
  Relational Operator9/1 -> AND3/2
  Relational Operator11/1 -> SR_Latch4/2
  SR_Latch5/1 -> [VVMC_LDW2ndTrigged_flg]  "VVMC_LDW2ndTrigged_flg"
  Constant34/1 -> Timer5/3
  Detect Decrease3/1 -> SR_Latch5/1
  Constant33/1 -> Timer4/3
  Constant36/1 -> Timer6/3
  [VVMC_LDWRest2Trigged_flg] -> Unit Delay10/1
  Unit Delay11/1 -> NOT11/1
  SR_Latch6/1 -> [VVMC_LDWRest2Trigged_flg]  "VVMC_LDWRest2Trigged_flg"
  NOT11/1 -> AND1/4
  NOT10/1 -> Timer6/2
  [VINP_IVISWCVibModeSta_enum] -> Switch2/3
  AND1/1 -> SR_Latch3/1
  Detect Increase5/1 -> AND4/1
  Constant32/1 -> Relational Operator12/2, Timer5/4
  AND2/1 -> SR_Latch7/2
  Unit Delay7/1 -> NOT7/1, Timer5/1
  [VVMC_LDWRestTrigged_flg] -> Detect Decrease3/1
  [VVMC_LDW2ndTrigged_flg] -> Unit Delay9/1
  [VVMC_LDWRest2Trigged_flg] -> Unit Delay12/1
  Detect Increase3/1 -> OR4/5
  [VVMC_LDW1stTrigged_flg] -> Detect Decrease2/1
  Detect Decrease5/1 -> AND2/1, SR_Latch7/1
  Unit Delay13/1 -> AND2/2
  Relational Operator12/1 -> SR_Latch5/2
  Unit Delay9/1 -> NOT9/1
  Constant30/1 -> Timer3/3
  Unit Delay10/1 -> Timer6/1, NOT10/1
  Constant37/1 -> Relational Operator9/2
  AND4/1 -> OR4/3
  Detect Decrease4/1 -> SR_Latch6/1
  Detect Decrease2/1 -> SR_Latch4/1
  [VVMC_LDW1stTrigged_flg] -> OR3/1
  [VVMC_LDW2ndTrigged_flg] -> Detect Decrease4/1
  Constant8/1 -> Detect Increase2/1
  Constant26/1 -> Timer4/4, Relational Operator11/2
  Switch3/1 -> Switch2/1
  [VVMC_LDWRestTrigged_flg] -> Unit Delay6/1
  NOT5/1 -> Timer3/2
  Unit Delay12/1 -> Detect Decrease5/1
  Constant31/1 -> Timer6/4, Relational Operator7/2
  Constant5/1 -> Relational Operator10/2
  Constant38/1 -> Switch2/2
  Detect Increase2/1 -> OR4/4
  NOT9/1 -> AND1/3
  Detect Increase4/1 -> AND3/1
  [VVMC_LDWRestTrigged_flg] -> Unit Delay8/1
  NOT6/1 -> Timer4/2
  Unit Delay5/1 -> NOT5/1, Timer3/1
  Relational Operator8/1 -> SR_Latch3/2
  [VINP_ADASLDWSta_enum] -> Relational Operator9/1, Detect Increase4/1  "VVMC_ADASLDWSta_enum"
  Timer5/1 -> Relational Operator12/1
  Unit Delay8/1 -> NOT8/1
  OR3/1 -> Switch3/2
  [VVMC_LDW2ndTrigged_flg] -> OR3/2
  Constant35/1 -> Switch3/3
  [VVMC_LDWRest2Trigged_flg] -> Unit Delay11/1
  NOT8/1 -> AND1/2
  AND3/1 -> OR4/2
  OR4/1 -> AND1/1  "LDWActTrigger"
  VINP_IVISWCVibModeSta_enum/1 -> [VINP_IVISWCVibModeSta_enum]
  [VINP_IVISWCVibModeSta_enum] -> Cast To Single/1
  Detect Change/1 -> AND5/1
  Cast To Single/1 -> Relational Operator5/1, Detect Change/1
  Relational Operator5/1 -> AND5/2
  Constant2/1 -> Relational Operator5/2
  AND5/1 -> OR4/1
  VDDM_VMCLatCtrlProhibited_flg/1 -> [VDDM_VMCLatCtrlProhibited_flg]
  [VDDM_VMCLatCtrlProhibited_flg] -> Switch10/2
  Constant12/1 -> Switch10/1
  Logical Operator1/1 -> Switch10/3
  VDDM_VMCLongCtrlProhibited_flg/1 -> [VDDM_VMCLongCtrlProhibited_flg]
  NOT/1 -> Logical Operator3/2
  [VDDM_VMCLongCtrlProhibited_flg] -> NOT/1
  Logical Operator3/1 -> Cast To Boolean/1
  [VDDM_VMCLongCtrlProhibited_flg] -> Switch1/2
  u2 > 0 (2)/1 -> Switch1/3
  Constant13/1 -> Switch1/1
